simulink model "rtwdemo_symbols"  (Simulink 6.0)
settings: Solver=ode3  StartTime=0.0  StopTime=10.0  RelTol=1e-3
libraries: rtwdemowidgets x1
settings Model: Creator=The MathWorks Inc.  LastModifiedBy=batserve  ExtModeAutoUpdateStatusClock=off
settings DataIOCC: SaveOutput=off  SaveTime=off
settings OptimizationCC: InlineParams=on  EnforceIntegerDowncast=off  StateBitsets=on  DataBitsets=on  UseTempVars=on  ZeroExternalMemoryAtStartup=off  ZeroInternalMemoryAtStartup=off  InitFltsAndDblsToZero=off  NoFixptDivByZeroProtection=on  OptimizeModelRefInitCode=on  LifeSpan=1
settings DebuggingCC: CheckExecutionContextPreStartOutputMsg=on  CheckExecutionContextRuntimeOutputMsg=on
settings RTWCC: SystemTargetFile=ert.tlc  TemplateMakefile=ert_default_tmf  Description=RTW Embedded Coder (no auto configuration)  GenerateReport=on  RTWVerbose=off  ProcessScript=ert_make_rtw_hook  IncludeHyperlinkInReport=on  LaunchReport=on
settings CodeAppCC: ForceParamTrailComments=on  IgnoreCustomStorageClasses=off  MaxIdLength=40  SimulinkDataObjDesc=on  InsertBlockDesc=on
settings ERTTargetCC: TargetFcnLib=ansi_tfl_tmw.mat  GenFloatMathFcnCalls=ANSI_C  GenerateSampleERTMain=on  IncludeMdlTerminateFcn=off  SupportNonFinite=off  SupportComplex=off  SupportContinuousTime=on  SupportNonInlinedSFcns=on  InlinedParameterPlacement=NonHierarchical  RootIOFormat=Individual Arguments  ERTCustomFileTemplate=example_file_process.tlc  InitialValueSource=Model

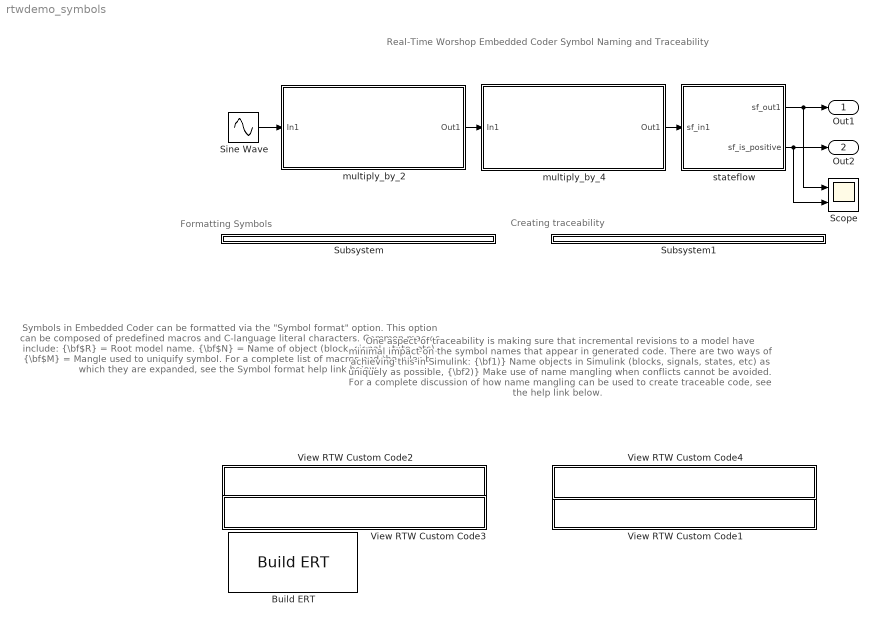
== system rtwdemo_symbols ==
  note: Real-Time Worshop Embedded Coder
      | Symbol Naming and Traceability
  note: Formatting Symbols
  note: Creating traceability
  note: Symbols in Embedded Coder can be formatted via
      | the "Symbol format" option. This option can be
      | composed of predefined macros and C-language
      | literal characters.
      |
      | Common macros include:
      |    {\bf$R} = Root model name.
      |    {\bf$N} = Name of object (block, signal, state, etc).
      |    {\bf$M} = Mangle used to uniquify symbol.
      |
      | For a complete list of macros and the rules by which
      | they are expanded, see the Symbol format help link
      | below.
  note: One aspect of traceability is making sure that
      | incremental revisions to a model have minimal
      | impact on the symbol names that appear in
      | generated code.  There are two ways of
      | achieving this in Simulink:
      |
      |   {\bf1)} Name objects in Simulink (blocks, signals,
      |        states, etc) as uniquely as possible,
      |   {\bf2)} Make use of name mangling when conflicts
      |        cannot be avoided.
      |
      | For a complete discussion of how name mangling
      | can be used to create traceable code, see the help
      | link below.
  Build ERT : rtwdemowidgets/Build ERT  attrib_overrides={'CustomSymbolStr'}
  Scope : Scope  NumInputPorts=2
      settings: YMin=-500~0  YMax=500~1
  Sine Wave : Sin  SineType=Sample based  Amplitude=100  SampleTime=.01
  Subsystem : Subsystem  PropExecContextAcrossSSBoundary=on
  Subsystem1 : Subsystem  PropExecContextAcrossSSBoundary=on
  View RTW Custom Code1 : Subsystem  PropExecContextAcrossSSBoundary=on
      mask init:
      | pos    = get_param(gcb, 'Position');
      | width  = pos(3) - pos(1);
      | height = pos(4) - pos(2);
      | 
      | 
      | % Compute arrow coordinates
      | arrowW = width  / 20;
      | arrowH = height / 2.5;
      | arrowX = width  / 50;
      | arrowY = height / 3;
      | arrowXvec = [arrowX, arrowX, arrowX + arrowW];
      | arrowYvec = [arrowY, arrowY + arrowH, arrowY + arrowH / 2];
      | 
      | % Compute text position
      | textXbuff = width / 30;
      | textX  = arrowX + arrowW + textXbuff;
      | textY  = height / 2;
      settings: OpenFcn=helpview([docroot '/mapfiles/ecoder_ug.map'], 'symbols_traceability')
      mask Display:
      | patch(arrowXvec, arrowYvec);
      | text(textX, textY, 'Double-click to view traceability help');
  View RTW Custom Code2 : Subsystem  PropExecContextAcrossSSBoundary=on
      mask init: same as rtwdemo_symbols/View RTW Custom Code1
      settings: OpenFcn=|
      | slCfgPrmDlg(bdroot,'Open');
      | slCfgPrmDlg(bdroot,'TurnToPage','Real-Time Workshop/Symbols');
      mask Display:
      | patch(arrowXvec, arrowYvec);
      | text(textX, textY, 'Double-click to view symbol format');
  View RTW Custom Code3 : Subsystem  PropExecContextAcrossSSBoundary=on
      mask init: same as rtwdemo_symbols/View RTW Custom Code1
      settings: OpenFcn=helpview([docroot '/mapfiles/ecoder_ug.map'], 'symbols_pane')
      mask Display:
      | patch(arrowXvec, arrowYvec);
      | text(textX, textY, 'Double-click to view symbol format help');
  View RTW Custom Code4 : Subsystem  PropExecContextAcrossSSBoundary=on
      mask init: same as rtwdemo_symbols/View RTW Custom Code1
      settings: OpenFcn=|
      | slCfgPrmDlg(bdroot,'Open');
      | slCfgPrmDlg(bdroot,'TurnToPage','Real-Time Workshop/Symbols');
      mask Display:
      | patch(arrowXvec, arrowYvec);
      | text(textX, textY, 'Double-click to view mangle settings');
  multiply_by_2 : Subsystem  TreatAsAtomicUnit=on  PropExecContextAcrossSSBoundary=on
      settings: RTWSystemCode=Function
      mask Display: fprintf('This atomic subsystem will\ngenerate a function of the form\n<model name>_<block name>\nwhich expands to\n%s_%s ',get_param(bdroot(gcbh),'name'),get_param(gcbh,'name'))
  multiply_by_4 : Subsystem  TreatAsAtomicUnit=on  PropExecContextAcrossSSBoundary=on
      settings: RTWSystemCode=Function  RTWFcnNameOpts=Use subsystem name
      mask Display: fprintf('This atomic subsystem will\ngenerate a function of the form\n<model name>_<block name>\nwhich expands to\n%s_%s ',get_param(bdroot(gcbh),'name'),get_param(gcbh,'name'))
  stateflow : Stateflow chart  PropExecContextAcrossSSBoundary=on
  Out1 : Outport
  Out2 : Outport  Port=2
  wires:
  Sine Wave/1 -> multiply_by_2/1(In1)
  multiply_by_2/1(Out1) -> multiply_by_4/1(In1)
  stateflow/1(sf_out1) -> Out1/1, Scope/1
  multiply_by_4/1(Out1) -> stateflow/1(sf_in1)
  stateflow/2(sf_is_positive) -> Out2/1, Scope/2

== system rtwdemo_symbols/Subsystem ==

== system rtwdemo_symbols/Subsystem1 ==

== system rtwdemo_symbols/View RTW Custom Code1 ==

== system rtwdemo_symbols/View RTW Custom Code2 ==

== system rtwdemo_symbols/View RTW Custom Code3 ==

== system rtwdemo_symbols/View RTW Custom Code4 ==

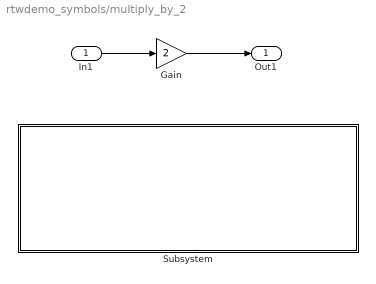
== system rtwdemo_symbols/multiply_by_2 ==
  In1 : Inport  Port=1  LatchInput=off
  Gain : Gain  Gain=2
  Subsystem : Subsystem  PropExecContextAcrossSSBoundary=on
      settings: OpenFcn=open_system('rtwdemo_symbols/multiply_by_4')
      mask Display: fprintf('The gain block in this subsystem will generate\na symbol named "Gain".  This will collide with\nthe symbol generated for the gain block in\n"rtwdemo_symbols/multiply_by_4/Gain".\n\n (double-click to open colliding block)')
  Out1 : Outport
  wires:
  In1/1 -> Gain/1
  Gain/1 -> Out1/1

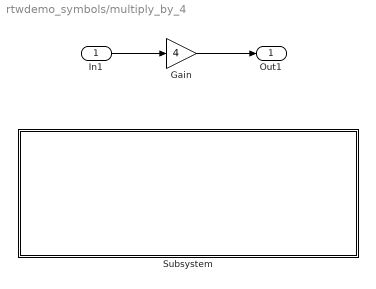
== system rtwdemo_symbols/multiply_by_4 ==
  In1 : Inport  Port=1  LatchInput=off
  Gain : Gain  Gain=4
  Subsystem : Subsystem  PropExecContextAcrossSSBoundary=on
      settings: OpenFcn=open_system('rtwdemo_symbols/multiply_by_2')
      mask Display: fprintf('The gain block in this subsystem will generate\na symbol named "Gain".  This will collide with\nthe symbol generated for the gain block in\n"rtwdemo_symbols/multiply_by_2/Gain".\n\n (double-click to open colliding block)')
  Out1 : Outport
  wires:
  In1/1 -> Gain/1
  Gain/1 -> Out1/1

== system rtwdemo_symbols/multiply_by_2/Subsystem ==

== system rtwdemo_symbols/multiply_by_4/Subsystem ==

== stateflow chart stateflow ==
  state positive_state
    entry:
    sf_is_positive = 1;
    sf_out1 = sf_in1;
  state negative_state
    entry:
    sf_is_positive = 0;
    sf_out1 = sf_in1;
  state result = sf_is_positive(val) [function]
    (default) -> (junction 7)
    (junction 7) -> (junction 8) : [val > 0]
        | {result = 1;}
    (junction 10) -> (junction 9) : {result = 0;}
    (junction 7) -> (junction 10)
  note: Note:
      | For demonstration purposes, inlining has been
      | turned off for this graphical function.  As a result,
      | a seperate c-code function will be generated that
      | respects the Real-Time Workshop naming rules.
  (default) -> positive_state
  positive_state -> negative_state : [~sf_is_positive(sf_in1)]
  negative_state -> positive_state : [sf_is_positive(sf_in1)]
  data: result function_output double size=1; val function_input double size=1; sf_in1 input inherited; sf_out1 output double size=1; sf_is_positive output double size=1
